simulink model "eval_longitudinal_ctrl_accel"  (R2019b)
settings: Solver=FixedStepDiscrete  StartTime=0.0  StopTime=inf  RelTol=1e-3  EnableMultiTasking=on
libraries: SCANeR_API x2
settings Model: Creator=sphilippe  LastModifiedBy=lpfeffer
settings DataIOCC: LimitDataPoints=on  SaveFormat=Array  ReturnWorkspaceOutputs=off
settings OptimizationCC: LifeSpan=inf
settings DebuggingCC: UnderspecifiedInitializationDetection=Classic  MergeDetectMultiDrivingBlocksExec=none  SolverPrmCheckMsg=warning  SFUnexpectedBacktrackingDiag=warning  SFNoUnconditionalDefaultTransitionDiag=warning  SFExecutionAtInitializationDiag=none  ArithmeticOperatorsInVariantConditions=warning
settings HardwareCC: ProdBitPerPointer=32  ProdBitPerSizeT=32  ProdBitPerPtrDiffT=32  ProdLargestAtomicFloat=None  ProdIntDivRoundTo=Undefined  ProdEndianess=Unspecified  ProdWordSize=32  ProdHWDeviceType=32-bit Generic
settings ModelReferenceCC: PropagateSignalLabelsOutOfModel=off
settings SFSimCC: SimUseLocalCustomCode=off  CustomCodeUndefinedFunction=UseInterfaceOnly
settings RTWCC: Description=SCANeR API Real-Time Target  SystemTargetFile=grt_scanerapi.tlc  TemplateMakefile=grt_scanerapi_vc.tmf  RTWUseLocalCustomCode=off
settings CodeAppCC: StateflowObjectComments=on
settings STFCustomTargetCC: GeneratePreprocessorConditionals=Disable all  MatFileLogging=on  CPPClassGenCompliant=on  GRTInterface=on  SystemTargetFile=grt_scanerapi.tlc
settings GRTTargetCC: TargetLangStandard=C89/C90 (ANSI)  ParMdlRefBuildCompliant=off  CompOptLevelCompliant=off  ConcurrentExecutionCompliant=off  GeneratePreprocessorConditionals=Disable all  CombineOutputUpdateFcns=off  GRTInterface=on  UseToolchainInfoCompliant=off
settings ConfigComp: CovMetricSettings=dw  CovHtmlReporting=on  CovSaveCumulativeToWorkspaceVar=on  CovSaveSingleToWorkspaceVar=on  CovExternalEMLEnable=off

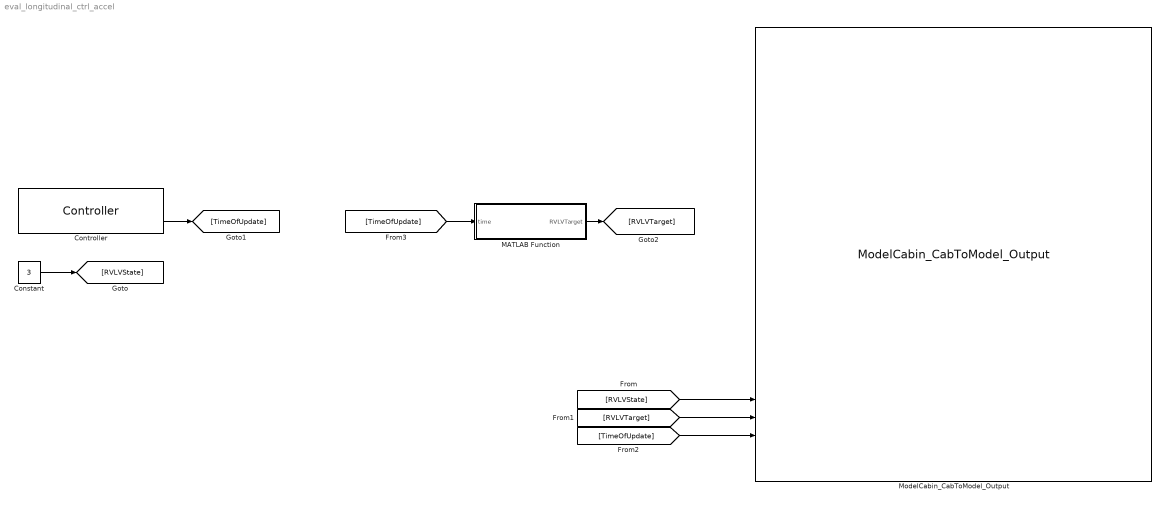
== system eval_longitudinal_ctrl_accel ==
  Constant : Constant  Value=3
  Controller : SCANeR_API/Controller  Priority=1  Config='SAMPLE_2022_LONGI_CTRL'  ProcName='LONGI_SIMULINK'  Frequency=100  NetworkOutputFrequency=10  TimeOut=30  IsSynchronized=off
      settings: SourceProductName=SCANeR API
  MATLAB Function : MATLAB Function  TreatAsAtomicUnit=on
  ModelCabin_CabToModel_Output : SCANeR_API/SHM outputs/ModelCabin/ModelCabin_CabToModel_Output  Priority=2  shmId=0
      settings: SourceProductName=SCANeR API
  wires:
  Constant/1 -> [RVLVState]
  [RVLVState] -> ModelCabin_CabToModel_Output/21
  [RVLVTarget] -> ModelCabin_CabToModel_Output/22
  Controller/2 -> [TimeOfUpdate]
  [TimeOfUpdate] -> ModelCabin_CabToModel_Output/23
  [TimeOfUpdate] -> MATLAB Function/1(time)
  MATLAB Function/1(RVLVTarget) -> [RVLVTarget]

== matlab function eval_longitudinal_ctrl_accel/MATLAB Function ==
  data: time input; RVLVTarget output
function RVLVTarget = fcn(time)
%#codegen

if (time < 10)
    RVLVTarget = 1.1;
else
    if (time < 20)
        RVLVTarget = 0;
    else
        RVLVTarget = -1.1;
    end
end
